simulink model "Hardware_With_Enhanced_Lead_Compensator"  (R2024b)
settings: Solver=FixedStepDiscrete  StartTime=0.0  StopTime=60  FixedStep=0.01  RelTol=1e-3  EnableMultiTasking=on
libraries: arduinolib x3, simulink x1
settings Model: ExtModeTrigDuration=2  Creator=mafur  LastModifiedBy=mafur
settings SolverCC: AutoInsertRateTranBlk=on
settings OptimizationCC: EnhancedBackFolding=on  PassReuseOutputArgsAs=Individual arguments  ZeroExternalMemoryAtStartup=off  ZeroInternalMemoryAtStartup=off  MaxStackSize=64  OptimizeBlockOrder=speed  DifferentSizesBufferReuse=on  OptimizationCustomize=off  EfficientTunableParamExpr=on
settings DebuggingCC: ParameterTunabilityLossMsg=error
settings HardwareCC: ProdBitPerPointer=32  ProdBitPerSizeT=32  ProdBitPerPtrDiffT=32  ProdLargestAtomicInteger=Long  ProdLargestAtomicFloat=Double  ProdWordSize=32  ProdHWDeviceType=ARM Compatible->ARM Cortex
settings SFSimCC: MATLABDynamicMemAlloc=off
settings RTWCC: Description=Embedded Coder  SystemTargetFile=ert.tlc  HardwareBoard=ESP32-WROOM(Arduino Compatible)  TLCOptions="-aInlineSetEventsForThisBaseRateFcn=TLC_FALSE -aSuppressMultiTaskScheduler=TLC_FALSE  -aRateBasedStepFcn=0"  TemplateMakefile=ert_default_tmf  Toolchain=ESP32  BuildConfiguration=Faster Runs
settings CodeAppCC: ForceParamTrailComments=on  IgnoreCustomStorageClasses=off  OperatorAnnotations=on  SimulinkDataObjDesc=on  SFDataObjDesc=on  InsertBlockDesc=on
settings ERTTargetCC: SupportContinuousTime=on  SupportVariableSizeSignals=on  ExtModeTransport=3  ExtModeStaticAlloc=on  ExtModeAutomaticAllocSize=off  ExtModeStaticAllocSize=65536  ExtModeMexFile=ext_xcp  ExtModeIntrfLevel=Level2 - Open  InlinedParameterPlacement=Hierarchical

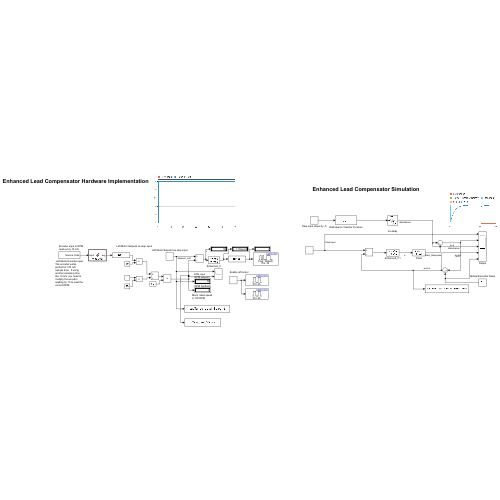
[thumbnail: Simulink's stored preview of the top-level diagram]
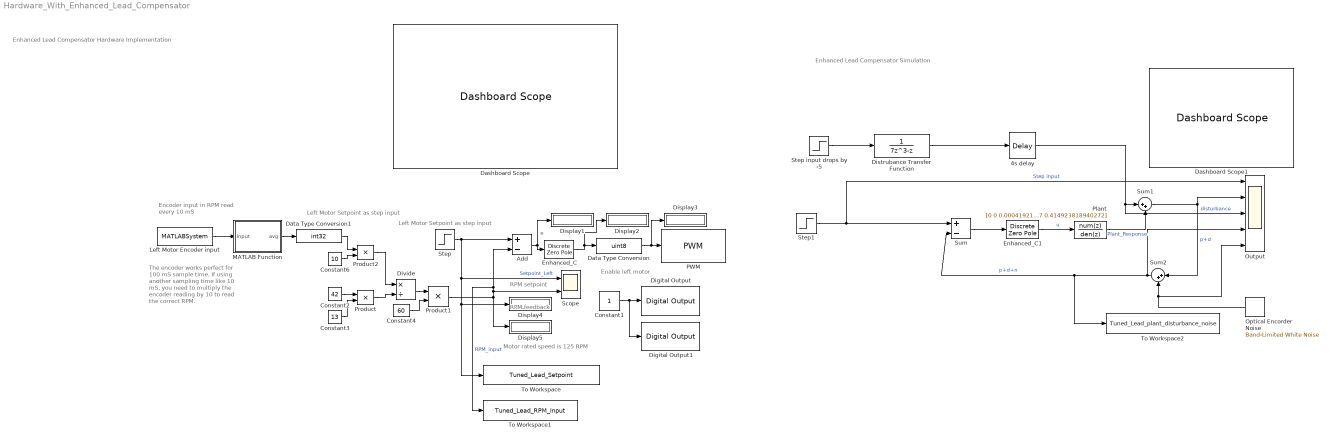
== system Hardware_With_Enhanced_Lead_Compensator ==
  note: Enhanced Lead Compensator Simulation
  note: RPM setpoint
  note: Left Motor Setpoint as step input
  note: Left Motor Setpoint as step input
  note: Motor rated speed is 125 RPM
  note: Enable left motor
  note: The encoder works perfect for 100 mS sample time. If using another sampling time like 10 mS, you need to multiply the encoder reading by 10 to read the correct RPM.
  note: Encoder input in RPM read every 10 mS
  note: RPM feedback
  note: Enhanced Lead Compensator Hardware Implementation
  " 4s delay" : TransportDelay  DelayTime=40
  Add : Sum  Inputs=+-
  Constant1 : Constant
  Constant2 : Constant  Value=42
  Constant3 : Constant  Value=13
  Constant4 : Constant  Value=60
  Constant6 : Constant  Value=10
  Dashboard Scope : DashboardScope
  Dashboard Scope1 : DashboardScope
  Data Type Conversion : DataTypeConversion  OutDataTypeStr=uint8  SaturateOnIntegerOverflow=off  RndMeth=Floor
  Data Type Conversion1 : DataTypeConversion  OutDataTypeStr=int32  SaturateOnIntegerOverflow=off  RndMeth=Floor
  Digital Output : arduinolib/Digital Output  pinNumber=25  Direction=output  blockPlatform=arduino
      settings: SourceProductName=Common
  Digital Output1 : arduinolib/Digital Output  pinNumber=26  Direction=output  blockPlatform=arduino
      settings: SourceProductName=Common
  Display{1..5} (5 alike) : Display
  Distrubance Transfer Function : DiscreteTransferFcn  Denominator=[7 0 -1 0]
  Divide : Product  Inputs=*/
  Enhanced_C : DiscreteZeroPole  Zeros=[0.8857]  Poles=[1]  Gain=3.2778  SampleTime=-1
  Enhanced_C1 : DiscreteZeroPole  Zeros=[0.8857]  Poles=[1]  Gain=3.2778  SampleTime=-1
  Left Motor Encoder input : MATLABSystem  System=EncoderRead  pinA=int8(36)  pinB=int8(39)  id=int8(0)  SampleTime=0.01
      mask Type: EncoderRead
      mask Display:
      | disp('Source');
      | port_label('output',1,'ticks');
  MATLAB Function : MATLAB Function  TreatAsAtomicUnit=on
  Optical Encorder Noise : simulink/Sources/Band-Limited White Noise  Cov=[0.000]  Ts=0.1  seed=[23341]
  Output : Scope  NumInputPorts=5
  PWM : arduinolib/PWM  pinNumber=32  frequencyType=Default  desiredFrequency=490.2  achievableFrequency=490.2
      settings: SourceProductName=Common
  Plant : DiscreteTransferFcn  Numerator=[0 0 0.000419217442677415]  Denominator=[1 -1.33793894475627 0.414923818940272]  SampleTime=0.01
  Product : Product
  Product1 : Product
  Product2 : Product
  Scope : Scope  NumInputPorts=2
  Step : Step  Time=0.5  After=50  SampleTime=0
  Step input drops by -5 : Step  After=-5  SampleTime=0
  Step1 : Step  After=10  SampleTime=0
  Sum : Sum  Inputs=+-
  Sum1 : Sum  Inputs=|++
  Sum2 : Sum  Inputs=|++
  To Workspace : ToWorkspace  VariableName=Tuned_Lead_Setpoint  SaveFormat=Structure With Time  SampleTime=-1
  To Workspace1 : ToWorkspace  VariableName=Tuned_Lead_RPM_Input  SaveFormat=Structure With Time  SampleTime=-1
  To Workspace2 : ToWorkspace  VariableName=Tuned_Lead_plant_disturbance_noise  SaveFormat=Structure With Time  SampleTime=-1
  wires:
  Enhanced_C/1 -> Display2/1, Data Type Conversion/1
  Constant2/1 -> Product/1
  Data Type Conversion1/1 -> Product2/1
  Step/1 -> Add/1, To Workspace/1, Display4/1, Scope/1  "Setpoint_Left"
  Product1/1 -> Display5/1, To Workspace1/1, Add/2, Scope/2  "RPM_input"
  Add/1 -> Enhanced_C/1, Display1/1  "e"
  Left Motor Encoder input/1 -> MATLAB Function/1(input)
  Constant3/1 -> Product/2
  Constant4/1 -> Product1/2
  Divide/1 -> Product1/1
  Product2/1 -> Divide/1
  Constant6/1 -> Product2/2
  Constant1/1 -> Digital Output1/1, Digital Output/1
  Product/1 -> Divide/2
  Data Type Conversion/1 -> Display3/1, PWM/1
  MATLAB Function/1(avg) -> Data Type Conversion1/1
  Optical Encorder Noise/1 -> Output/5, Sum2/2
  Plant/1 -> Sum1/2  "Plant_Response"
  Step input drops by -5/1 -> Distrubance Transfer Function/1
  Step1/1 -> Sum/1, Output/1  "Step input"
  Sum1/1 -> Sum2/1, Output/2  "p+d"
  Sum2/1 -> Sum/2, To Workspace2/1, Output/4  "p+d+n"
  Enhanced_C1/1 -> Plant/1  "u"
  " 4s delay"/1 -> Sum1/1, Output/3  "disturbance"
  Sum/1 -> Enhanced_C1/1
  Distrubance Transfer Function/1 -> " 4s delay"/1

== matlab function Hardware_With_Enhanced_Lead_Compensator/MATLAB Function ==
  data: input input; avg output
function avg = ringBuffer(input)
    % Define persistent variables
    persistent buffer index sum count;
    if isempty(buffer)
        buffer = zeros(1, 10); % Initialize buffer with 10 zeros
        index = 1; % Initialize index
        sum = 0; % Initialize sum
        count = 0; % Initialize count
    end
    
    % Update the buffer
    sum = sum - buffer(index); % Subtract the old value from sum
    new_input = double(input);
    buffer(index) = new_input; % Insert the new value
    sum = sum + new_input; % Add the new value to sum
    
    % Update the index
    index = index + 1;
    if index > 10
        index = 1; % Wrap around the index
    end
    
    % Update the count
    if  count < 10
        count = count + 1;
    end
    
    % Calculate the average
     avg = sum / count;
end
